simulink model "safety"  (R2018b)
settings: Solver=FixedStepDiscrete  StartTime=0.0  StopTime=10.0  RelTol=1e-3
settings Model: ExtModeTrigDuration=2  Creator=sin29  LastModifiedBy=sin29
settings OptimizationCC: DefaultParameterBehavior=Inlined  UseDivisionForNetSlopeComputation=on  UseFloatMulNetSlope=on  InlineInvariantSignals=on  PassReuseOutputArgsAs=Individual arguments  ZeroExternalMemoryAtStartup=off  ZeroInternalMemoryAtStartup=off  NoFixptDivByZeroProtection=on  EfficientFloat2IntCast=on  LifeSpan=1  MaxStackSize=64  OptimizeBlockOrder=speed  DifferentSizesBufferReuse=on
settings DebuggingCC: ParameterTunabilityLossMsg=error
settings HardwareCC: ProdBitPerInt=16  ProdBitPerPointer=16  ProdBitPerSizeT=16  ProdBitPerPtrDiffT=16  ProdLargestAtomicFloat=None  ProdWordSize=8  ProdLongLongMode=on  ProdHWDeviceType=Atmel->AVR
settings SFSimCC: MATLABDynamicMemAlloc=off
settings RTWCC: SystemTargetFile=ert.tlc  HardwareBoard=Arduino Uno  TemplateMakefile=ert_default_tmf  GenerateReport=on  Toolchain=Arduino AVR  BuildConfiguration=Faster Runs  IncludeHyperlinkInReport=on  LaunchReport=on  GenerateTraceInfo=on  GenerateTraceReport=on  GenerateTraceReportSl=on  GenerateTraceReportSf=on  GenerateTraceReportEml=on  GenerateCodeMetricsReport=on
settings CodeAppCC: ForceParamTrailComments=on  IgnoreCustomStorageClasses=off  OperatorAnnotations=on  SimulinkDataObjDesc=on  SFDataObjDesc=on  CustomSymbolStrGlobalVar=rt$N$M  CustomSymbolStrType=$N$M  CustomSymbolStrFcn=$N$M$F  CustomSymbolStrMacro=$N$M  InsertBlockDesc=on
settings ERTTargetCC: IncludeMdlTerminateFcn=off  CombineSignalStateStructs=on  SupportAbsoluteTime=off  SupportComplex=off  SupportNonInlinedSFcns=on  InlinedParameterPlacement=NonHierarchical  ERTFilePackagingFormat=CompactWithDataFile

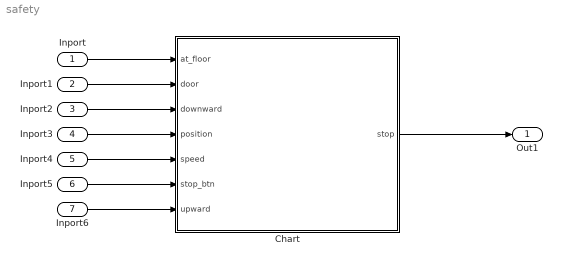
== system safety ==
  Inport : Inport
  Inport1 : Inport  Port=2
  Inport2 : Inport  Port=3
  Inport3 : Inport  Port=4
  Inport4 : Inport  Port=5
  Inport5 : Inport  Port=6
  Inport6 : Inport  Port=7
  Chart : Stateflow chart  TreatAsAtomicUnit=on
  Out1 : Outport
  wires:
  Inport/1 -> Chart/1(at_floor)
  Inport1/1 -> Chart/2(door)
  Inport2/1 -> Chart/3(downward)
  Inport3/1 -> Chart/4(position)
  Inport4/1 -> Chart/5(speed)
  Inport5/1 -> Chart/6(stop_btn)
  Inport6/1 -> Chart/7(upward)
  Chart/1(stop) -> Out1/1

== stateflow chart safety/Chart ==
  state down_stop
    entry :
    stop = 1;
  state both_dir_stop
    entry:
    stop = 1;
  state monitor
    during:
    stop = 0;
  state door_stop
    entry :
    stop = 1;
  state stop_button
    entry :
    stop = 1;
  state speed_stop
    entry :
    stop = 1;
  state top_stop
    entry :
    stop = 1;
  down_stop -> down_stop [order 1] : [after (10, msec) && position == 800 && at_floor == -1 && upward == 1]
  down_stop -> monitor [order 2] : [after (10, msec)  &&( at_floor ~= -1 || downward == 0)]
  monitor -> down_stop [order 5] : [after (10, msec) && position == 0 && at_floor == -1 && downward == 1]
  (default) -> monitor
  both_dir_stop -> both_dir_stop [order 2] : [after(10, msec) && upward == 1 && downward == 1]
  both_dir_stop -> monitor [order 1] : [after(10, msec) && (upward == 0 || downward == 0)]
  monitor -> both_dir_stop [order 6] : [after(10, msec) && upward == 1 && downward == 1]
  monitor -> top_stop [order 3] : [after (10, msec) && position == 800 && at_floor == -1 && upward == 1]
  monitor -> door_stop [order 1] : [after(10, msec) && door == 1 && at_floor ==-1]
  door_stop -> monitor [order 2] : [after(3, msec) && door == 0]
  top_stop -> monitor [order 1] : [after (10, msec)  &&( at_floor ~= -1 || upward == 0)]
  monitor -> stop_button [order 2] : [after (10, msec) && stop_btn == 1]
  stop_button -> monitor [order 2] : [after(3, msec) && stop_btn == 0]
  speed_stop -> monitor [order 1] : [after (10, msec) && speed <= 50]
  monitor -> speed_stop [order 4] : [after (10, msec) && speed > 50]
  door_stop -> door_stop [order 1] : [after(3, msec) && door == 1]
  stop_button -> stop_button [order 1] : [after(3, msec) && stop_btn == 1]
  speed_stop -> speed_stop [order 2] : [after (10, msec) && speed > 50]
  top_stop -> top_stop [order 2] : [after (10, msec) && position == 800 && at_floor == -1 && upward == 1]
  data: at_floor input; door input; downward input; position input; speed input; stop_btn input; upward input; stop output
